simulink model "KD_cl_harness_cl_ouports_added"  (R2015b)
settings: Solver=ode45  StartTime=0  StopTime=inf  FixedStep=0.01  MaxStep=0.005  RelTol=1e-5  AbsTol=1e-5
undefined symbols (not defined in the file or in its folder): A2, bin_vec, c_0, c_1000, c_1000inv, c_100inv, c_1d2p4, c_1p7, c_4400inv, c_5500inv, c_80, c_compmap, c_ctok, c_fflow_max, c_fflow_min, c_filt, c_flowdiv, c_flowmin, c_flowmult, c_inf, c_km1d2k, c_n1, c_p00001, c_p01, c_p1e9, c_p4d1p4, c_pincomp, c_rair, c_roacorr, c_rpmtoradpers, c_svrthrottle1, c_svrthrottle2, c_svrthrottlearg, c_svrthrottlebeta, c_vnliftmax, c_vnliftmin, cl_offset, clff, Coefs, const, const_exhat, const_vec, Dual_array, dual_zero, egr_ecu_ff, expcon, f_mat, gs_jul, HQP_eps, HQP_INF, HQP_saturation, IV, L2, length_L, maxL, mHQP_saturation, minL, Newton, nRed, num_constraints ... (+22)
libraries: simulink x33
(part 1 of 6)
settings Model: Creator=spolavarapu  LastModifiedBy=rthekkal
settings SolverCC: ZeroCrossControl=DisableAll
settings DataIOCC: LimitDataPoints=off  SaveFormat=StructureWithTime  SignalLoggingSaveFormat=ModelDataLogs  SaveOutput=off  SignalLogging=off  DSMLogging=off  SaveTime=off
settings OptimizationCC: BlockReduction=off  OptimizeBlockIOStorage=off  BufferReuse=off  GlobalBufferReuse=off  ExpressionFolding=off  ExpressionDepthLimit=2147483647  LocalBlockOutputs=off  EfficientFloat2IntCast=on  OptimizeModelRefInitCode=on
settings DebuggingCC: SignalInfNanChecking=error  SignalRangeChecking=error  ReadBeforeWriteMsg=DisableAll  WriteAfterWriteMsg=DisableAll  WriteAfterReadMsg=DisableAll  AlgebraicLoopMsg=error  ArtificialAlgebraicLoopMsg=error  SaveWithDisabledLinksMsg=error  SaveWithParameterizedLinksMsg=error  UnderspecifiedInitializationDetection=Classic  MergeDetectMultiDrivingBlocksExec=none  CheckExecutionContextPreStartOutputMsg=on  CheckExecutionContextRuntimeOutputMsg=on  BlockPriorityViolationMsg=error  SolverPrmCheckMsg=error  InheritedTsInSrcMsg=error  MultiTaskDSMMsg=none  SigSpecEnsureSampleTimeMsg=error  CheckMatrixSingularityMsg=error  IntegerOverflowMsg=error  ParameterUnderflowMsg=error  ParameterPrecisionLossMsg=error  ParameterTunabilityLossMsg=error  UnderSpecifiedDataTypeMsg=warning  UnnecessaryDatatypeConvMsg=warning  VectorMatrixConversionMsg=error  FcnCallInpInsideContextMsg=EnableAllAsWarning  SignalLabelMismatchMsg=warning  UnconnectedInputMsg=error  UnconnectedOutputMsg=error  UnconnectedLineMsg=error  SFcnCompatibilityMsg=error  UniqueDataStoreMsg=error  BusObjectLabelMismatch=error  RootOutportRequireBusObject=error  AssertControl=DisableAll  ModelReferenceIOMsg=error  ModelReferenceIOMismatchMessage=error  UnknownTsInhSupMsg=error  ModelReferenceDataLoggingMessage=error  StateNameClashWarn=warning  StrictBusMsg=ErrorOnBusTreatedAsVector  IntegerSaturationMsg=error
settings HardwareCC: ProdBitPerPointer=32  ProdLargestAtomicFloat=None  ProdIntDivRoundTo=Undefined  ProdEndianess=Unspecified  ProdWordSize=32  ProdHWDeviceType=32-bit Generic
settings RTWCC: SystemTargetFile=ert.tlc  TemplateMakefile=ert_default_tmf  Description=Real-Time Workshop Embedded Coder
settings CodeAppCC: ForceParamTrailComments=on  IgnoreCustomStorageClasses=off  MangleLength=4  CustomSymbolStrType=$N$R$M  InternalIdentifier=Classic  ReqsInCode=on
settings ERTTargetCC: GenerateSampleERTMain=on  IncludeMdlTerminateFcn=off  GeneratePreprocessorConditionals=Disable all  SuppressErrorStatus=on  SupportAbsoluteTime=off  SupportNonFinite=off  ParenthesesLevel=Maximum  ERTCustomFileTemplate=example_file_process.tlc  PreserveExpressionOrder=on  PreserveIfCondition=on
settings ConfigComp: CovModelRefEnable=Off

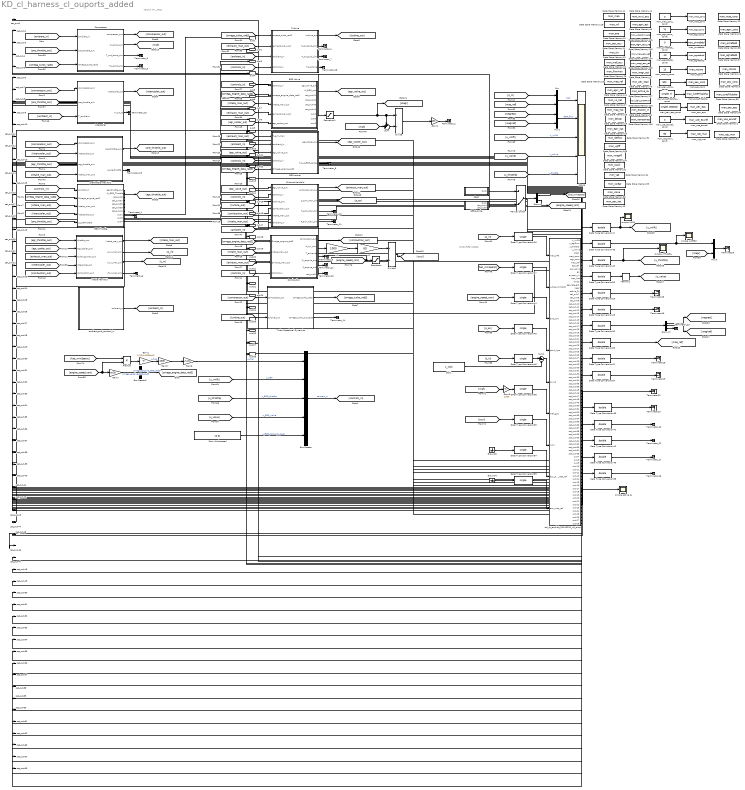
== system KD_cl_harness_cl_ouports_added ==
  note: Version A4 _ 0611
  note: SIMPLIFIED MODEL
  Bus Creator : BusCreator  Inputs=5
  Bus Creator2 : BusCreator  Inputs=1
  Combsution : Subsystem
  Compressor : Subsystem
  Data Store Memory10 : DataStoreMemory  DataStoreName=mon_ene  ReadBeforeWriteMsg=warning  WriteAfterWriteMsg=warning  WriteAfterReadMsg=warning  InitialValue=1  OutDataTypeStr=single
  Data Store Memory100 : DataStoreMemory  DataStoreName=mon_remapmap  ReadBeforeWriteMsg=warning  WriteAfterWriteMsg=warning  WriteAfterReadMsg=warning  OutDataTypeStr=single
  Data Store Memory103 : DataStoreMemory  DataStoreName=mon_egrr_ecu_ref  ReadBeforeWriteMsg=warning  WriteAfterWriteMsg=warning  WriteAfterReadMsg=warning  InitialValue=1  OutDataTypeStr=single
  Data Store Memory104 : DataStoreMemory  DataStoreName=mon_map_ecu_ref  ReadBeforeWriteMsg=warning  WriteAfterWriteMsg=warning  WriteAfterReadMsg=warning  InitialValue=1  OutDataTypeStr=single
  Data Store Memory105 : DataStoreMemory  DataStoreName=mon_wegr_ecu_ref  ReadBeforeWriteMsg=warning  WriteAfterWriteMsg=warning  WriteAfterReadMsg=warning  InitialValue=1  OutDataTypeStr=single
  Data Store Memory106 : DataStoreMemory  DataStoreName=mon_wtpostinverse  ReadBeforeWriteMsg=warning  WriteAfterWriteMsg=warning  WriteAfterReadMsg=warning  InitialValue=1  OutDataTypeStr=single
  Data Store Memory107 : DataStoreMemory  DataStoreName=mon_vwegrff  ReadBeforeWriteMsg=warning  WriteAfterWriteMsg=warning  WriteAfterReadMsg=warning  InitialValue=1  OutDataTypeStr=single
  Data Store Memory108 : DataStoreMemory  DataStoreName=mon_vgtff  ReadBeforeWriteMsg=warning  WriteAfterWriteMsg=warning  WriteAfterReadMsg=warning  InitialValue=1  OutDataTypeStr=single
  Data Store Memory11 : DataStoreMemory  DataStoreName=mon_pex_ecu  ReadBeforeWriteMsg=warning  WriteAfterWriteMsg=warning  WriteAfterReadMsg=warning  InitialValue=1  OutDataTypeStr=single
  Data Store Memory118 : DataStoreMemory  DataStoreName=mon_wf  ReadBeforeWriteMsg=warning  WriteAfterWriteMsg=warning  WriteAfterReadMsg=warning  InitialValue=1  OutDataTypeStr=single
  Data Store Memory126 : DataStoreMemory  DataStoreName=mon_delU_HQPKWIK  ReadBeforeWriteMsg=warning  WriteAfterWriteMsg=warning  WriteAfterReadMsg=warning  InitialValue=[0;0;0]  OutDataTypeStr=single
  Data Store Memory127 : DataStoreMemory  DataStoreName=mon_active_SL  ReadBeforeWriteMsg=warning  WriteAfterWriteMsg=warning  WriteAfterReadMsg=warning  OutDataTypeStr=int32
  Data Store Memory13 : DataStoreMemory  DataStoreName=mon_tin  ReadBeforeWriteMsg=warning  WriteAfterWriteMsg=warning  WriteAfterReadMsg=warning  InitialValue=1  OutDataTypeStr=single
  Data Store Memory14 : DataStoreMemory  DataStoreName=man_ntcons  ReadBeforeWriteMsg=warning  WriteAfterWriteMsg=warning  WriteAfterReadMsg=warning  InitialValue=15  OutDataTypeStr=single
  Data Store Memory2 : DataStoreMemory  DataStoreName=man_use_ecuref  ReadBeforeWriteMsg=warning  WriteAfterWriteMsg=warning  WriteAfterReadMsg=warning  OutDataTypeStr=single
  Data Store Memory20 : DataStoreMemory  DataStoreName=mon_maf_ecu  ReadBeforeWriteMsg=warning  WriteAfterWriteMsg=warning  WriteAfterReadMsg=warning  InitialValue=1  OutDataTypeStr=single
  Data Store Memory21 : DataStoreMemory  DataStoreName=man_map_cons  ReadBeforeWriteMsg=warning  WriteAfterWriteMsg=warning  WriteAfterReadMsg=warning  OutDataTypeStr=single
  Data Store Memory22 : DataStoreMemory  DataStoreName=man_egrr_cons  ReadBeforeWriteMsg=warning  WriteAfterWriteMsg=warning  WriteAfterReadMsg=warning  InitialValue=70  OutDataTypeStr=single
  Data Store Memory23 : DataStoreMemory  DataStoreName=mon_map_ref  ReadBeforeWriteMsg=warning  WriteAfterWriteMsg=warning  WriteAfterReadMsg=warning  InitialValue=1  OutDataTypeStr=single
  Data Store Memory24 : DataStoreMemory  DataStoreName=mon_egrr_ref  ReadBeforeWriteMsg=warning  WriteAfterWriteMsg=warning  WriteAfterReadMsg=warning  InitialValue=1  OutDataTypeStr=single
  Data Store Memory25 : DataStoreMemory  DataStoreName=mon_map_hat  ReadBeforeWriteMsg=warning  WriteAfterWriteMsg=warning  WriteAfterReadMsg=warning  InitialValue=1  OutDataTypeStr=single
  Data Store Memory26 : DataStoreMemory  DataStoreName=mon_egrr_hat  ReadBeforeWriteMsg=warning  WriteAfterWriteMsg=warning  WriteAfterReadMsg=warning  InitialValue=1  OutDataTypeStr=single
  Data Store Memory27 : DataStoreMemory  DataStoreName=mon_x1_hat  ReadBeforeWriteMsg=warning  WriteAfterWriteMsg=warning  WriteAfterReadMsg=warning  InitialValue=zeros(nRed,1)  OutDataTypeStr=single
  Data Store Memory28 : DataStoreMemory  DataStoreName=mon_flowmax  ReadBeforeWriteMsg=warning  WriteAfterWriteMsg=warning  WriteAfterReadMsg=warning  InitialValue=1  OutDataTypeStr=single
  Data Store Memory29 : DataStoreMemory  DataStoreName=mon_delvgt  ReadBeforeWriteMsg=warning  WriteAfterWriteMsg=warning  WriteAfterReadMsg=warning  InitialValue=1  OutDataTypeStr=single
  Data Store Memory31 : DataStoreMemory  DataStoreName=mon_delflow  ReadBeforeWriteMsg=warning  WriteAfterWriteMsg=warning  WriteAfterReadMsg=warning  InitialValue=1  OutDataTypeStr=single
  Data Store Memory32 : DataStoreMemory  DataStoreName=mon_slack  ReadBeforeWriteMsg=warning  WriteAfterWriteMsg=warning  WriteAfterReadMsg=warning  InitialValue=1  OutDataTypeStr=single
  Data Store Memory34 : DataStoreMemory  DataStoreName=mon_vgt  ReadBeforeWriteMsg=warning  WriteAfterWriteMsg=warning  WriteAfterReadMsg=warning  InitialValue=1  OutDataTypeStr=single
  Data Store Memory35 : DataStoreMemory  DataStoreName=mon_uwegr  ReadBeforeWriteMsg=warning  WriteAfterWriteMsg=warning  WriteAfterReadMsg=warning  InitialValue=1  OutDataTypeStr=single
  Data Store Memory36 : DataStoreMemory  DataStoreName=mon_valve  ReadBeforeWriteMsg=warning  WriteAfterWriteMsg=warning  WriteAfterReadMsg=warning  InitialValue=1  OutDataTypeStr=single
  Data Store Memory37 : DataStoreMemory  DataStoreName=man_egrrefadd  ReadBeforeWriteMsg=warning  WriteAfterWriteMsg=warning  WriteAfterReadMsg=warning  InitialValue=-10  OutDataTypeStr=single
  Data Store Memory38 : DataStoreMemory  DataStoreName=man_pinrefadd  ReadBeforeWriteMsg=warning  WriteAfterWriteMsg=warning  WriteAfterReadMsg=warning  OutDataTypeStr=single
  Data Store Memory41 : DataStoreMemory  DataStoreName=mon_map  ReadBeforeWriteMsg=warning  WriteAfterWriteMsg=warning  WriteAfterReadMsg=warning  InitialValue=1  OutDataTypeStr=single
  Data Store Memory43 : DataStoreMemory  DataStoreName=mon_pex_hat  ReadBeforeWriteMsg=warning  WriteAfterWriteMsg=warning  WriteAfterReadMsg=warning  InitialValue=3  OutDataTypeStr=single
  Data Store Memory44 : DataStoreMemory  DataStoreName=mon_wcyl_ecu  ReadBeforeWriteMsg=warning  WriteAfterWriteMsg=warning  WriteAfterReadMsg=warning  InitialValue=1  OutDataTypeStr=single
  Data Store Memory46 : DataStoreMemory  DataStoreName=mon_egrr_est  ReadBeforeWriteMsg=warning  WriteAfterWriteMsg=warning  WriteAfterReadMsg=warning  InitialValue=1  OutDataTypeStr=single
  Data Store Memory47 : DataStoreMemory  DataStoreName=mon_wegr_est  ReadBeforeWriteMsg=warning  WriteAfterWriteMsg=warning  WriteAfterReadMsg=warning  InitialValue=1  OutDataTypeStr=single
  Data Store Memory54 : DataStoreMemory  DataStoreName=man_pex_eps  ReadBeforeWriteMsg=warning  WriteAfterWriteMsg=warning  WriteAfterReadMsg=warning  InitialValue=single(.000002)  OutDataTypeStr=single
  Data Store Memory78 : DataStoreMemory  DataStoreName=mon_pex_lead  ReadBeforeWriteMsg=warning  WriteAfterWriteMsg=warning  WriteAfterReadMsg=warning  OutDataTypeStr=single
  Data Store Memory84 : DataStoreMemory  DataStoreName=man_vgt_max  ReadBeforeWriteMsg=warning  WriteAfterWriteMsg=warning  WriteAfterReadMsg=warning  InitialValue=90  OutDataTypeStr=single
  Data Store Memory85 : DataStoreMemory  DataStoreName=man_tuneFiltalpha  ReadBeforeWriteMsg=warning  WriteAfterWriteMsg=warning  WriteAfterReadMsg=warning  InitialValue=single(.7)  OutDataTypeStr=single
  Data Store Memory9 : DataStoreMemory  DataStoreName=man_pex_cons  ReadBeforeWriteMsg=warning  WriteAfterWriteMsg=warning  WriteAfterReadMsg=warning  InitialValue=300  OutDataTypeStr=single
  Data Store Memory91 : DataStoreMemory  DataStoreName=mon_expcon_in  ReadBeforeWriteMsg=warning  WriteAfterWriteMsg=warning  WriteAfterReadMsg=warning  InitialValue=zeros(nRed+12,1)  OutDataTypeStr=single
  Data Type Conversion{26,35,37..38,44..46,53..54} (9 alike) : DataTypeConversion  OutDataTypeStr=single
  Data Type Conversion{28..31,33..34,39,41..43,47..50,55} (15 alike) : DataTypeConversion  OutDataTypeStr=double
  Demux : Demux  Outputs=2
  Demux2 : Demux  Outputs=3
  Divide : Product  Inputs=*/
  Divide1 : Product  Inputs=*/
  EGR Throttle : Subsystem
  EGR Valve : Subsystem
  EGR cooler : Subsystem
  Exhaust Manifold : Subsystem
  From Workspace4 : FromWorkspace  VariableName=[0 3]  SampleTime=0  Interpolate=off  OutputAfterFinalValue=Holding final value
  Gain1 : Gain  Gain=1/(120/4/832e-9)
  Gain2 : Gain  Gain=100
  Gain5 : Gain  Gain=1000
  Gain6 : Gain  Gain=1/1000
  Gain7 : Gain  Gain=pi/30
  Gain9 : Gain  Gain=1000
  Ground3 : Ground
  Ground4 : Ground
  Intake Manifold : Subsystem
  Intercooler : Subsystem
  Manual Switch : ManualSwitch  CurrentSetting=0
  Memory1 : Memory
  Mux : Mux  Inputs=2
  Mux1 : Mux  Inputs=2
  Mux3 : Mux  Inputs=2
  NEDC_cycle : Subsystem
  Product : Product  RndMeth=Zero
  Saturation : Saturate  UpperLimit=6000  LowerLimit=500
  Saturation1 : Saturate  UpperLimit=inf  LowerLimit=0
      settings: AttributesFormatString=%<LowerLimit>\n%<UpperLimit>
  Scope : Scope  NumInputPorts=5
  Sum : Sum  Inputs=++|
  Sum1 : Sum  Inputs=|+-
  Terminator{5,12..13,15..16,18..19} (7 alike) : Terminator
  Terminator_{1..9,11,13..23,26} (22 alike) : Terminator
  Turbine : Subsystem
  Turbo Rotational Dynamics : Subsystem
  ambient_and_controls_in : Subsystem
  ctok1 : Constant  Value=c_ctok  OutDataTypeStr=single  SampleTime=sample_time
      settings: AttributesFormatString=%<Value>\n%<SampleTime>
  ctrl_rb_explicit_20140220_v6_simp : Subsystem  TreatAsAtomicUnit=on  SystemSampleTime=sample_time
  man_egrr_cons : DataStoreWrite  DataStoreName=man_egrr_cons
  man_egrr_cons_const : Constant  Value=70  OutDataTypeStr=single
  man_egrrefadd : DataStoreWrite  DataStoreName=man_egrrefadd
  man_egrrefadd_const : Constant  Value=-10  VectorParams1D=off  OutDataTypeStr=single
      settings: AttributesFormatString=%<VectorParams1D>
  man_map_cons : DataStoreWrite  DataStoreName=man_map_cons
  man_map_cons_const : Constant  Value=0  OutDataTypeStr=single
  man_ntcons : DataStoreWrite  DataStoreName=man_ntcons
  man_ntcons_const : Constant  Value=15  OutDataTypeStr=single
  man_pex_cons : DataStoreWrite  DataStoreName=man_pex_cons
  man_pex_cons_const : Constant  Value=300  OutDataTypeStr=single
  man_pex_eps : DataStoreWrite  DataStoreName=man_pex_eps
  man_pex_eps_const : Constant  Value=single(.000002)  OutDataTypeStr=single
  man_pinrefadd : DataStoreWrite  DataStoreName=man_pinrefadd
  man_pinrefadd_const : Constant  Value=0  OutDataTypeStr=single
  man_tuneFiltalpha : DataStoreWrite  DataStoreName=man_tuneFiltalpha
  man_tuneFiltalpha_const : Constant  Value=single(.7)  OutDataTypeStr=single
  man_use_ecuref : DataStoreWrite  DataStoreName=man_use_ecuref
  man_use_ecuref_const : Constant  Value=0  OutDataTypeStr=single
  man_vgt_max : DataStoreWrite  DataStoreName=man_vgt_max
  man_vgt_max_const : Constant  Value=90  OutDataTypeStr=single
  n1 : Gain  Gain=1000
      settings: AttributesFormatString=%<Gain>
  n2 : Gain  Gain=60
      settings: AttributesFormatString=%<Gain>
  pre-throttle manifold : Subsystem
  simple VNlift : Scope
  simple active SL : Scope
  simple uThrottle : Scope
  simple uWEGR : Scope
  steps : Subsystem
  sat_out-1 : Outport
  sat_out-2 : Outport  Port=2
  sat_out-3 : Outport  Port=3
  sat_out-4 : Outport  Port=4
  sat_out-5 : Outport  Port=5
  sat_out-6 : Outport  Port=6
  sat_out-7 : Outport  Port=7
  sat_out-8 : Outport  Port=8
  sat_out-9 : Outport  Port=9
  sat_out-10 : Outport  Port=10
  sat_out-11 : Outport  Port=11
  sat_out-12 : Outport  Port=12
  sat_out-13 : Outport  Port=13
  sat_out-14 : Outport  Port=14
  sat_out-15 : Outport  Port=15
  sat_out-16 : Outport  Port=16
  sat_out-17 : Outport  Port=17
  sat_out-18 : Outport  Port=18
  sat_out-19 : Outport  Port=19
  sat_out-20 : Outport  Port=20
  sat_out-21 : Outport  Port=21
  sat_out-22 : Outport  Port=22
  sat_out-23 : Outport  Port=23
  sat_out-24 : Outport  Port=24
  sat_out-25 : Outport  Port=25
  sat_out-26 : Outport  Port=26
  sat_out-27 : Outport  Port=27
  sat_out-28 : Outport  Port=28
  sat_out-29 : Outport  Port=29
  sat_out-30 : Outport  Port=30
  sat_out-31 : Outport  Port=31
  sat_out-32 : Outport  Port=32
  sat_out-33 : Outport  Port=33
  sat_out-34 : Outport  Port=34
  sat_out-35 : Outport  Port=35
  sat_out-36 : Outport  Port=36
  sat_out-37 : Outport  Port=37
  sat_out-38 : Outport  Port=38
  sat_out-39 : Outport  Port=39
  sat_out-40 : Outport  Port=40
  sat_out-41 : Outport  Port=41
  sat_out-42 : Outport  Port=42
  sat_out-43 : Outport  Port=43
  sat_out-44 : Outport  Port=44
  sat_out-45 : Outport  Port=45
  sat_out-46 : Outport  Port=46
  sat_out-47 : Outport  Port=47
  sat_out-48 : Outport  Port=48
  sat_out-49 : Outport  Port=49
  sat_out-50 : Outport  Port=50
  sat_out-51 : Outport  Port=51
  sat_out-52 : Outport  Port=52
  sat_out-53 : Outport  Port=53
  sat_out-54 : Outport  Port=54
  sat_out-55 : Outport  Port=55
  sat_out-56 : Outport  Port=56
  sat_out-57 : Outport  Port=57
  sat_out-58 : Outport  Port=58
  sat_out-59 : Outport  Port=59
  sat_out-60 : Outport  Port=60
  sat_out-61 : Outport  Port=61
  sat_out-62 : Outport  Port=62
  sat_out-63 : Outport  Port=63
  sat_out-64 : Outport  Port=64
  sat_out-65 : Outport  Port=65
  out-1 : Outport  Port=66
  out-2 : Outport  Port=67
  out-3 : Outport  Port=68
  out-4 : Outport  Port=69
  out-5 : Outport  Port=70
  out-6 : Outport  Port=71
  out-7 : Outport  Port=72
  out-8 : Outport  Port=73
  out-9 : Outport  Port=74
  out-10 : Outport  Port=75
  out-11 : Outport  Port=76
  out-12 : Outport  Port=77
  out-13 : Outport  Port=78
  out-14 : Outport  Port=79
  out-15 : Outport  Port=80
  out-16 : Outport  Port=81
  out-17 : Outport  Port=82
  out-18 : Outport  Port=83
  out-19 : Outport  Port=84
  out-20 : Outport  Port=85
  out-21 : Outport  Port=86
  out-22 : Outport  Port=87
  out-23 : Outport  Port=88
  out-24 : Outport  Port=89
  out-25 : Outport  Port=90
  out-26 : Outport  Port=91
  out-27 : Outport  Port=92
  out-28 : Outport  Port=93
  wires:
  ambient_and_controls_in/1(ambient_in) -> [ambient_in]
  Compressor/1(compressor_out) -> [compressor_out]
  Intercooler/1(intercooler_out) -> [intercooler_out]
  EGR Throttle/1(egr_throttle_out) -> [egr_throttle_out]
  Intake Manifold/1(intake_man_out) -> [intake_man_out]
  Turbine/1(turbine_out) -> [turbine_out]
  EGR Valve/1(egr_valve_out) -> [egr_valve_out]
  EGR cooler/1(egr_cooler_out) -> [egr_cooler_out]
  Exhaust Manifold/1(exhaust_man_out) -> [exhaust_man_out]
  Combsution/1(combustion_out) -> [combustion_out]
  pre-throttle manifold/1(pre_throttle_out) -> [pre_throttle_out]
  Compressor/2(W_comp_sim) -> [maf]
  Compressor/3(T_out_comp_sim) -> Terminator_3/1
  Compressor/4(Tq_comp_sim) -> Terminator_5/1
  EGR Valve/2(W_EGR_out) -> Saturation1/1, sat_out-2/1
  Exhaust Manifold/4(F_exh_man_sim) -> Terminator_11/1
  Intake Manifold/3(T_in_man_sim) -> [t_in]
  Intercooler/2(T_out_IC) -> Terminator_15/1
  Turbine/4(Tq_turbine) -> Terminator_18/1
  pre-throttle manifold/2(p_pre_throttle) -> Terminator_19/1
  Turbo Rotational Dynamics/1(Omega_turbo_radS) -> [omega_turbo_radS]
  Combsution/4(W_engine_out) -> Terminator_21/1
  Combsution/5(F_engine_out) -> Terminator_20/1
  Intake Manifold/2(p_in_man_sim) -> [p_in]
  Turbo Rotational Dynamics/2(Omega_turbo_out_radS) -> Terminator_14/1
  [maf] -> Sum/2
  Sum/1 -> Divide/2
  Divide/1 -> Gain2/1
  Exhaust Manifold/2(p_exh_man_sim) -> [p_ex]
  Turbine/2(W_out_turb_sim) -> Terminator_4/1
  Turbine/3(T_out_turb_sim) -> Terminator_7/1
  [p_in] -> Mux/1
  [u_vnlift] -> Bus Creator/2  "u_VGT"
  [u_throttle] -> Bus Creator/3  "u_EGR_throttle"
  [u_valve] -> Bus Creator/4  "u_EGR_valve"
  From Workspace4/1 -> Bus Creator/5  "u_EGR_cooler_bypass"
  Bus Creator/1 -> [controls_in]  "controls_in"
  Bus Creator2/1 -> [omega_engine_data_radS]  "omega_engine_data_radS"
  Mux/1 -> Scope/1  "MAP"
  Mux1/1 -> Scope/2  "EGR_flow"
  [map_ref] -> Mux/2
  Gain2/1 -> Terminator_2/1
  Exhaust Manifold/3(T_exh_man_sim) -> Terminator_16/1
  Gain7/1 -> Bus Creator2/1  "omega_engine_data_radS"
  [engine_speed_rpm] -> Gain7/1, Product/2
  [u_vnlift] -> Scope/3  "u_vnlift"
  [u_valve] -> Scope/4  "u_valve"
  EGR Throttle/2(W_EGR_Throttle) -> Terminator_1/1
  Saturation1/1 -> Sum/1, Divide/1, [Wegr]
  [ambient_in] -> Compressor/1(ambient_in)
  [compressor_out] -> Intercooler/1(compressor_out)
  [compressor_out] -> pre-throttle manifold/1(compressor_out)
  [intercooler_out] -> pre-throttle manifold/2(intercooler_out)
  [egr_throttle_out] -> pre-throttle manifold/3(egr_throttle_out)
  [controls_in] -> EGR Throttle/1(controls_in)
  [omega_engine_data_radS] -> EGR Throttle/2(Omega_engine_radS)
  [intake_man_out] -> EGR Throttle/3(intake_man_out)
  [intercooler_out] -> EGR Throttle/4(intercooler_out)
  [egr_throttle_out] -> Intake Manifold/1(throttle_out)
  [egr_cooler_out] -> Intake Manifold/2(egr_cooler_out)
  [exhaust_man_out] -> Intake Manifold/3(exhaust_man_out)
  [omega_turbo_radS] -> Compressor/3(Omega_turbo_radS)
  [pre_throttle_out] -> Compressor/2(pre_throttle_out)
  [pre_throttle_out] -> Intercooler/2(pre_throttle_out)
  [intercooler_out] -> Intake Manifold/4(intecooler_out)
  [combustion_out] -> Intake Manifold/5(combustion_out)
  [pre_throttle_out] -> EGR Throttle/5(p_preThrottle)
  [intake_man_out] -> pre-throttle manifold/4(Intake_man_out)
  [ambient_in] -> Intercooler/3(T_ambient)
  [omega_engine_data_radS] -> Combsution/1(Omega_engine_radS)
  [intake_man_out] -> Combsution/2(intake_man_out)
  [exhaust_man_out] -> Combsution/3(exhaust_man_out)
  [controls_in] -> Combsution/4(controls_in)
  [intake_man_out] -> Exhaust Manifold/5(intake_man_out)
  [egr_valve_out] -> Exhaust Manifold/1(egr_valve_out)
  [controls_in] -> Exhaust Manifold/2(controls_in)
  [turbine_out] -> Exhaust Manifold/3(turbine_out)
  [ambient_in] -> EGR cooler/2(ambient_in)
  [exhaust_man_out] -> EGR cooler/1(T_exh_man)
  [egr_valve_out] -> EGR cooler/3(egr_valve_out)
  [controls_in] -> EGR cooler/4(controls_in)
  [omega_engine_data_radS] -> EGR cooler/5(Omega_engine_radS)
  [exhaust_man_out] -> EGR Valve/4(exhaust_man_out)
  [controls_in] -> EGR Valve/1(controls_in)
  [omega_engine_data_radS] -> EGR Valve/2(omega_engine_data_radS)
  [intake_man_out] -> EGR Valve/3(intake_man_out)
  [omega_turbo_radS] -> Turbine/1(omega_turbo_radS)
  [exhaust_man_out] -> Turbine/2(exhaust_man_out)
  [ambient_in] -> Turbine/3(ambient_In)
  [controls_in] -> Turbine/4(controls_In)
  [compressor_out] -> Turbo Rotational Dynamics/1(compressor_out)
  [turbine_out] -> Turbo Rotational Dynamics/2(turbine_out)
  [combustion_out] -> Exhaust Manifold/4(combustion_out)
  [egr_cooler_out] -> EGR Valve/5(egr_cooler_out)
  [ambient_in] -> Exhaust Manifold/6(ambient_in)
  Intake Manifold/4(F_in_man_sim) -> Terminator_6/1
  Combsution/3(T_exhaust) -> Terminator_9/1
  Product/1 -> Gain1/1
  [fuel_mm3perst] -> Product/1
  [u_throttle] -> Scope/5  "u_throttle"
  NEDC_cycle/1(Out1) -> Manual Switch/2
  steps/1(Out1) -> Manual Switch/1
  Manual Switch/1 -> Demux/1
  Demux/1 -> [fuel_mm3perst]
  Demux/2 -> [engine_speed_rpm]
  EGR cooler/2(T_out_EGR_cooler) -> Terminator_8/1
  Gain5/1 -> Gain6/1
  Gain6/1 -> Bus Creator/1  "u_fuel"
  Gain1/1 -> Gain5/1  "u_fuel"
  Combsution/2(W_cyl_sim) -> n1/1
  n1/1 -> n2/1
  n2/1 -> Divide1/1
  [engine_speed_rpm] -> Saturation/1, sat_out-1/1
  Divide1/1 -> [wcyl]
  Saturation/1 -> Divide1/2
  ctrl_rb_explicit_20140220_v6_simp/3(u_throttle) -> Data Type Conversion49/1
  ctrl_rb_explicit_20140220_v6_simp/2(u_egrflow) -> Data Type Conversion48/1
  ctrl_rb_explicit_20140220_v6_simp/4(u_valve) -> Data Type Conversion50/1
  ctrl_rb_explicit_20140220_v6_simp/5(slack) -> Data Type Conversion28/1
  ctrl_rb_explicit_20140220_v6_simp/6(map_cons) -> Data Type Conversion29/1
  ctrl_rb_explicit_20140220_v6_simp/7(egr_cons) -> Data Type Conversion30/1
  ctrl_rb_explicit_20140220_v6_simp/1(u_vnlift) -> Data Type Conversion47/1
  [p_in] -> Data Type Conversion26/1
  [fuel_mm3perst] -> Data Type Conversion37/1
  [engine_speed_rpm] -> Data Type Conversion44/1
  [p_ex] -> Data Type Conversion45/1
  [t_in] -> Data Type Conversion46/1
  ctrl_rb_explicit_20140220_v6_simp/8(map_ref) -> Data Type Conversion33/1
  Data Type Conversion49/1 -> simple uThrottle/1, [u_throttle]
  Data Type Conversion50/1 -> Memory1/1
  Data Type Conversion28/1 -> Terminator15/1
  Data Type Conversion29/1 -> Terminator16/1
  Data Type Conversion30/1 -> Demux2/1
  Data Type Conversion33/1 -> [map_ref]
  ctrl_rb_explicit_20140220_v6_simp/9(egr_ref) -> Data Type Conversion31/1
  Data Type Conversion31/1 -> Terminator18/1
  ctrl_rb_explicit_20140220_v6_simp/10(pex_cons) -> Data Type Conversion34/1
  Data Type Conversion34/1 -> Terminator19/1
  Data Type Conversion48/1 -> Mux3/1, simple uWEGR/1
  Mux3/1 -> Terminator5/1
  [Wegr] -> Mux3/2
  ctrl_rb_explicit_20140220_v6_simp/11(gs) -> Terminator12/1
  Data Type Conversion26/1 -> ctrl_rb_explicit_20140220_v6_simp/1(map_kPa)
  Data Type Conversion37/1 -> ctrl_rb_explicit_20140220_v6_simp/2(u_fuel_mm3pst)
  Data Type Conversion44/1 -> ctrl_rb_explicit_20140220_v6_simp/3(ene_rpm)
  Data Type Conversion45/1 -> ctrl_rb_explicit_20140220_v6_simp/4(pexh_kpa)
  Memory1/1 -> [u_valve]
  Data Type Conversion39/1 -> Terminator13/1
  Gain9/1 -> Data Type Conversion38/1
  [maf] -> Gain9/1
  Data Type Conversion38/1 -> ctrl_rb_explicit_20140220_v6_simp/6(maf_gps)
  Data Type Conversion46/1 -> Sum1/1
  ctok1/1 -> Sum1/2
  Sum1/1 -> ctrl_rb_explicit_20140220_v6_simp/5(t_in_C)
  [wcyl] -> Data Type Conversion35/1
  Data Type Conversion35/1 -> ctrl_rb_explicit_20140220_v6_simp/7(wcyl)
  ctrl_rb_explicit_20140220_v6_simp/13(pex_hat) -> Data Type Conversion41/1
  ctrl_rb_explicit_20140220_v6_simp/14(dwdp) -> Data Type Conversion42/1
  Data Type Conversion42/1 -> Terminator_22/1
  Data Type Conversion41/1 -> Terminator_13/1
  ctrl_rb_explicit_20140220_v6_simp/15(egr_rate_est) -> Data Type Conversion43/1
  Data Type Conversion43/1 -> Terminator_17/1
  ctrl_rb_explicit_20140220_v6_simp/17(active_SL) -> simple active SL/1
  Demux2/3 -> Terminator_23/1
  Demux2/2 -> [wegrref]
  Demux2/1 -> [wegrest]
  Data Type Conversion47/1 -> simple VNlift/1, [u_vnlift]
  Data Type Conversion54/1 -> ctrl_rb_explicit_20140220_v6_simp/8(ecu_egr_rate_ref)
  Data Type Conversion53/1 -> ctrl_rb_explicit_20140220_v6_simp/9(ecu_map_ref)
  Ground3/1 -> Data Type Conversion54/1
  Ground4/1 -> Data Type Conversion53/1
  ctrl_rb_explicit_20140220_v6_simp/16(wegr) -> Data Type Conversion55/1
  Data Type Conversion55/1 -> Terminator_26/1
  ctrl_rb_explicit_20140220_v6_simp/12(expcon_in) -> Data Type Conversion39/1
  man_map_cons_const/1 -> man_map_cons/1
  man_egrr_cons_const/1 -> man_egrr_cons/1
  man_pinrefadd_const/1 -> man_pinrefadd/1
  man_egrrefadd_const/1 -> man_egrrefadd/1
  man_ntcons_const/1 -> man_ntcons/1
  man_pex_cons_const/1 -> man_pex_cons/1
  man_tuneFiltalpha_const/1 -> man_tuneFiltalpha/1
  man_pex_eps_const/1 -> man_pex_eps/1
  man_vgt_max_const/1 -> man_vgt_max/1
  man_use_ecuref_const/1 -> man_use_ecuref/1
  [wegrest] -> Mux1/1
  [wegrref] -> Mux1/2
  Combsution/6(sat_out-3) -> sat_out-3/1
  NEDC_cycle/2(sat_out-4) -> sat_out-4/1
  NEDC_cycle/3(sat_out-5) -> sat_out-5/1
  EGR Throttle/3(sat_out-6) -> sat_out-6/1
  ctrl_rb_explicit_20140220_v6_simp/18(sat_out-7) -> sat_out-7/1
  ctrl_rb_explicit_20140220_v6_simp/19(sat_out-8) -> sat_out-8/1
  ctrl_rb_explicit_20140220_v6_simp/20(sat_out-9) -> sat_out-9/1
  ctrl_rb_explicit_20140220_v6_simp/21(sat_out-10) -> sat_out-10/1
  ctrl_rb_explicit_20140220_v6_simp/22(sat_out-11) -> sat_out-11/1
  ctrl_rb_explicit_20140220_v6_simp/23(sat_out-12) -> sat_out-12/1
  ctrl_rb_explicit_20140220_v6_simp/24(sat_out-13) -> sat_out-13/1
  ctrl_rb_explicit_20140220_v6_simp/25(sat_out-14) -> sat_out-14/1
  ctrl_rb_explicit_20140220_v6_simp/26(sat_out-15) -> sat_out-15/1
  ctrl_rb_explicit_20140220_v6_simp/27(sat_out-16) -> sat_out-16/1
  ctrl_rb_explicit_20140220_v6_simp/28(sat_out-17) -> sat_out-17/1
  ctrl_rb_explicit_20140220_v6_simp/29(sat_out-18) -> sat_out-18/1
  ctrl_rb_explicit_20140220_v6_simp/30(sat_out-19) -> sat_out-19/1
  ctrl_rb_explicit_20140220_v6_simp/31(sat_out-20) -> sat_out-20/1
  ctrl_rb_explicit_20140220_v6_simp/32(sat_out-21) -> sat_out-21/1
  ctrl_rb_explicit_20140220_v6_simp/33(sat_out-22) -> sat_out-22/1
  ctrl_rb_explicit_20140220_v6_simp/34(sat_out-23) -> sat_out-23/1
  ctrl_rb_explicit_20140220_v6_simp/35(sat_out-24) -> sat_out-24/1
  ctrl_rb_explicit_20140220_v6_simp/36(sat_out-25) -> sat_out-25/1
  ctrl_rb_explicit_20140220_v6_simp/37(sat_out-26) -> sat_out-26/1
  ctrl_rb_explicit_20140220_v6_simp/38(sat_out-27) -> sat_out-27/1
  ctrl_rb_explicit_20140220_v6_simp/39(sat_out-28) -> sat_out-28/1
  ctrl_rb_explicit_20140220_v6_simp/40(sat_out-29) -> sat_out-29/1
  ctrl_rb_explicit_20140220_v6_simp/41(sat_out-30) -> sat_out-30/1
  ctrl_rb_explicit_20140220_v6_simp/42(sat_out-31) -> sat_out-31/1
  ctrl_rb_explicit_20140220_v6_simp/43(sat_out-32) -> sat_out-32/1
  ctrl_rb_explicit_20140220_v6_simp/44(sat_out-33) -> sat_out-33/1
  ctrl_rb_explicit_20140220_v6_simp/45(sat_out-34) -> sat_out-34/1
  ctrl_rb_explicit_20140220_v6_simp/46(sat_out-35) -> sat_out-35/1
  ctrl_rb_explicit_20140220_v6_simp/47(sat_out-36) -> sat_out-36/1
  EGR Throttle/4(sat_out-37) -> sat_out-37/1
  EGR Throttle/5(sat_out-38) -> sat_out-38/1
  EGR Throttle/6(sat_out-39) -> sat_out-39/1
  EGR Throttle/7(sat_out-40) -> sat_out-40/1
  EGR Valve/3(sat_out-41) -> sat_out-41/1
  EGR Valve/4(sat_out-42) -> sat_out-42/1
  EGR Valve/5(sat_out-43) -> sat_out-43/1
  EGR Valve/6(sat_out-44) -> sat_out-44/1
  ctrl_rb_explicit_20140220_v6_simp/48(sat_out-45) -> sat_out-45/1
  ctrl_rb_explicit_20140220_v6_simp/49(sat_out-46) -> sat_out-46/1
  ctrl_rb_explicit_20140220_v6_simp/50(sat_out-47) -> sat_out-47/1
  ctrl_rb_explicit_20140220_v6_simp/51(sat_out-48) -> sat_out-48/1
  ctrl_rb_explicit_20140220_v6_simp/52(sat_out-49) -> sat_out-49/1
  ctrl_rb_explicit_20140220_v6_simp/53(sat_out-50) -> sat_out-50/1
  ctrl_rb_explicit_20140220_v6_simp/54(sat_out-51) -> sat_out-51/1
  ctrl_rb_explicit_20140220_v6_simp/55(sat_out-52) -> sat_out-52/1
  ctrl_rb_explicit_20140220_v6_simp/56(sat_out-53) -> sat_out-53/1
  ctrl_rb_explicit_20140220_v6_simp/57(sat_out-54) -> sat_out-54/1
  ctrl_rb_explicit_20140220_v6_simp/58(sat_out-55) -> sat_out-55/1
  ctrl_rb_explicit_20140220_v6_simp/59(sat_out-56) -> sat_out-56/1
  ctrl_rb_explicit_20140220_v6_simp/60(sat_out-57) -> sat_out-57/1
  ctrl_rb_explicit_20140220_v6_simp/61(sat_out-58) -> sat_out-58/1
  ctrl_rb_explicit_20140220_v6_simp/62(sat_out-59) -> sat_out-59/1
  ctrl_rb_explicit_20140220_v6_simp/63(sat_out-60) -> sat_out-60/1
  ctrl_rb_explicit_20140220_v6_simp/64(sat_out-61) -> sat_out-61/1
  ctrl_rb_explicit_20140220_v6_simp/65(sat_out-62) -> sat_out-62/1
  ctrl_rb_explicit_20140220_v6_simp/66(sat_out-63) -> sat_out-63/1
  ctrl_rb_explicit_20140220_v6_simp/67(sat_out-64) -> sat_out-64/1
  ctrl_rb_explicit_20140220_v6_simp/68(sat_out-65) -> sat_out-65/1
  EGR Throttle/8(out-1) -> out-1/1
  EGR Valve/7(out-2) -> out-2/1
  EGR Throttle/9(out-3) -> out-3/1
  EGR Throttle/10(out-4) -> out-4/1
  EGR Valve/8(out-5) -> out-5/1
  EGR Valve/9(out-6) -> out-6/1
  ctrl_rb_explicit_20140220_v6_simp/69(out-7) -> out-7/1
  ctrl_rb_explicit_20140220_v6_simp/70(out-8) -> out-8/1
  ctrl_rb_explicit_20140220_v6_simp/71(out-9) -> out-9/1
  ctrl_rb_explicit_20140220_v6_simp/72(out-10) -> out-10/1
  ctrl_rb_explicit_20140220_v6_simp/73(out-11) -> out-11/1
  ctrl_rb_explicit_20140220_v6_simp/74(out-12) -> out-12/1
  ctrl_rb_explicit_20140220_v6_simp/75(out-13) -> out-13/1
  ctrl_rb_explicit_20140220_v6_simp/76(out-14) -> out-14/1
  ctrl_rb_explicit_20140220_v6_simp/77(out-15) -> out-15/1
  ctrl_rb_explicit_20140220_v6_simp/78(out-16) -> out-16/1
  ctrl_rb_explicit_20140220_v6_simp/79(out-17) -> out-17/1
  ctrl_rb_explicit_20140220_v6_simp/80(out-18) -> out-18/1
  ctrl_rb_explicit_20140220_v6_simp/81(out-19) -> out-19/1
  ctrl_rb_explicit_20140220_v6_simp/82(out-20) -> out-20/1
  ctrl_rb_explicit_20140220_v6_simp/83(out-21) -> out-21/1
  ctrl_rb_explicit_20140220_v6_simp/84(out-22) -> out-22/1
  ctrl_rb_explicit_20140220_v6_simp/85(out-23) -> out-23/1
  ctrl_rb_explicit_20140220_v6_simp/86(out-24) -> out-24/1
  ctrl_rb_explicit_20140220_v6_simp/87(out-25) -> out-25/1
  ctrl_rb_explicit_20140220_v6_simp/88(out-26) -> out-26/1
  ctrl_rb_explicit_20140220_v6_simp/89(out-27) -> out-27/1
  ctrl_rb_explicit_20140220_v6_simp/90(out-28) -> out-28/1

== system KD_cl_harness_cl_ouports_added/Combsution ==
  note: W_engine = W_cyl + u_fuel
  note: Gain block has no significance
      | just to add color to the lines
  Omega_engine_radS : Inport
  intake_man_out : Inport  Port=2
  exhaust_man_out : Inport  Port=3
  controls_in : Inport  Port=4
  Bus Creator : BusCreator  Inputs=4
  Bus Creator1 : BusCreator  Inputs=4
  Bus Selector : BusSelector  OutputSignals=controls_in.u_fuel,omega_engine_data_radS.omega_engine_data_radS,intake_man_out.p_in_man,exhaust_man_out.p_exh_man,intake_man_out.T_in_man,exhaust_man_out.T_exh_man
  Bus Selector1 : BusSelector  OutputSignals=controls_in.u_fuel,intake_man_out.F_in_man
  Bus Selector2 : BusSelector  OutputSignals=omega_engine_data_radS.omega_engine_data_radS,intake_man_out.T_in_man,controls_in.u_fuel,intake_man_out.F_in_man
  "Exhaust " : Subsystem
  Fcn : Fcn  Expr=(u(2)*u(3)+(1+14.6)*u(1))/(u(1)+u(3))
  Gain : Gain
  Mux : Mux  Inputs=3
  Saturation : Saturate  UpperLimit=1  LowerLimit=0
  Sum : Sum
  cylinder comp : Subsystem
  combustion_out : Outport
  W_cyl_sim : Outport  Port=2
  T_exhaust : Outport  Port=3
  W_engine_out : Outport  Port=4
  F_engine_out : Outport  Port=5
  sat_out-3 : Outport  Port=6
  wires:
  cylinder comp/1(W_cyl_sim) -> Gain/1  "W_cylinderr"
  "Exhaust "/1(T_exhaust) -> T_exhaust/1, Bus Creator/2  "T_exhaust"
  Bus Creator/1 -> combustion_out/1  "combustion_out"
  Omega_engine_radS/1 -> Bus Creator1/1
  intake_man_out/1 -> Bus Creator1/2
  exhaust_man_out/1 -> Bus Creator1/3
  controls_in/1 -> Bus Creator1/4
  Bus Creator1/1 -> Bus Selector/1, Bus Selector2/1, Bus Selector1/1
  Bus Selector/2 -> cylinder comp/1(omega_engine_radS)  "<omega_engine_data_radS>"
  Bus Selector/3 -> cylinder comp/2(p_intake_man)  "<p_in_man>"
  Bus Selector/4 -> cylinder comp/3(p_exhaust_man)  "<p_exh_man>"
  Bus Selector/5 -> cylinder comp/4(T_intake_man)  "<T_in_man>"
  Bus Selector/6 -> cylinder comp/5(T_exhaust_man)  "<T_exh_man>"
  Bus Selector2/1 -> "Exhaust "/1(omega_engine_radS)  "<omega_engine_data_radS>"
  Bus Selector2/3 -> "Exhaust "/4(u_fuel)  "<u_fuel>"
  Bus Selector2/4 -> "Exhaust "/5(F1_in_man)  "<F_in_man>"
  Bus Selector2/2 -> "Exhaust "/2(T_intake_man)  "<T_in_man>"
  Bus Selector/1 -> Sum/1  "<u_fuel>"
  Sum/1 -> W_engine_out/1, Bus Creator/4  "W_engine_out"
  Bus Selector1/1 -> Mux/1  "<u_fuel>"
  Bus Selector1/2 -> Mux/2  "<F_in_man>"
  Gain/1 -> "Exhaust "/3(W_cyl), Mux/3, Bus Creator/1, W_cyl_sim/1, Sum/2  "W_cylinder"
  Mux/1 -> Fcn/1
  Fcn/1 -> Saturation/1, sat_out-3/1  "F_engine_out1"
  Saturation/1 -> F_engine_out/1, Bus Creator/3  "F_engine_out"

== system KD_cl_harness_cl_ouports_added/Compressor ==
  ambient_in : Inport
  pre_throttle_out : Inport  Port=2
  Omega_turbo_radS : Inport  Port=3
  Bus Creator : BusCreator  Inputs=3
  Bus Creator1 : BusCreator  Inputs=3
  Bus Selector : BusSelector  OutputSignals=ambient_in.p_in_comp_data,pre_throttle_out.p_pre_throttle,ambient_in.T_in_comp_data,Omega_turbo_radS.Omega_turbo_radS
  Comp Map : Subsystem
  compressor_out : Outport
  W_comp_sim : Outport  Port=2
  T_out_comp_sim : Outport  Port=3
  Tq_comp_sim : Outport  Port=4
  wires:
  Comp Map/1(W_comp_sim) -> W_comp_sim/1, Bus Creator/1  "W_compressor"
  Comp Map/2(T_out_comp_sim) -> T_out_comp_sim/1, Bus Creator/2  "T_out_comp_sim"
  Bus Creator/1 -> compressor_out/1  "compressor_out"
  Comp Map/3(Tq_comp) -> Tq_comp_sim/1, Bus Creator/3  "Tq_comp_sim"
  ambient_in/1 -> Bus Creator1/1
  pre_throttle_out/1 -> Bus Creator1/2
  Omega_turbo_radS/1 -> Bus Creator1/3
  Bus Creator1/1 -> Bus Selector/1
  Bus Selector/1 -> Comp Map/1(p_in_comp)  "<p_in_comp_data>"
  Bus Selector/2 -> Comp Map/2(p_out_comp)  "<p_pre_throttle>"
  Bus Selector/3 -> Comp Map/3(T_in_comp_data)  "<T_in_comp_data>"
  Bus Selector/4 -> Comp Map/4(omega_turbo_data_radS)  "<Omega_turbo_radS>"

== system KD_cl_harness_cl_ouports_added/EGR Throttle ==
  controls_in : Inport
  Omega_engine_radS : Inport  Port=2
  intake_man_out : Inport  Port=3
  intercooler_out : Inport  Port=4
  p_preThrottle : Inport  Port=5
  Bus Creator : BusCreator  Inputs=1
  Bus Creator1 : BusCreator  Inputs=5
  Bus Selector : BusSelector  OutputSignals=controls_in.u_EGR_throttle,omega_engine_data_radS.omega_engine_data_radS,intake_man_out.p_in_man,intercooler_out.T_out_IC,pre_throttle_out.p_pre_throttle
  EGR Throttle : Subsystem
  egr_throttle_out : Outport
  W_EGR_Throttle : Outport  Port=2
  sat_out-6 : Outport  Port=3
  sat_out-37 : Outport  Port=4
  sat_out-38 : Outport  Port=5
  sat_out-39 : Outport  Port=6
  sat_out-40 : Outport  Port=7
  out-1 : Outport  Port=8
  out-3 : Outport  Port=9
  out-4 : Outport  Port=10
  wires:
  EGR Throttle/1(ThrottleFlow_kgpers) -> Bus Creator/1, W_EGR_Throttle/1  "W_EGR_Throttle"
  Bus Creator/1 -> egr_throttle_out/1  "egr_throttle_out"
  controls_in/1 -> Bus Creator1/1
  Omega_engine_radS/1 -> Bus Creator1/2
  intake_man_out/1 -> Bus Creator1/3
  intercooler_out/1 -> Bus Creator1/4
  Bus Creator1/1 -> Bus Selector/1
  Bus Selector/1 -> EGR Throttle/1(u_EGR_throttle)  "<u_EGR_throttle>"
  Bus Selector/2 -> EGR Throttle/2(omega_engine_radS)  "<omega_engine_data_radS>"
  Bus Selector/3 -> EGR Throttle/3(p_intake_man)  "<p_in_man>"
  Bus Selector/4 -> EGR Throttle/4(T_out_IC)  "<T_out_IC>"
  Bus Selector/5 -> EGR Throttle/5(p_preThrottle)  "<p_pre_throttle>"
  p_preThrottle/1 -> Bus Creator1/5
  EGR Throttle/2(sat_out-6) -> sat_out-6/1
  EGR Throttle/3(sat_out-37) -> sat_out-37/1
  EGR Throttle/4(sat_out-38) -> sat_out-38/1
  EGR Throttle/5(sat_out-39) -> sat_out-39/1
  EGR Throttle/6(sat_out-40) -> sat_out-40/1
  EGR Throttle/7(out-1) -> out-1/1
  EGR Throttle/8(out-3) -> out-3/1
  EGR Throttle/9(out-4) -> out-4/1

== system KD_cl_harness_cl_ouports_added/EGR Valve ==
  controls_in : Inport
  omega_engine_data_radS : Inport  Port=2
  intake_man_out : Inport  Port=3
  exhaust_man_out : Inport  Port=4
  egr_cooler_out : Inport  Port=5
  Bus Creator : BusCreator  Inputs=1
  Bus Creator1 : BusCreator  Inputs=5
  Bus Selector : BusSelector  OutputSignals=controls_in.u_EGR_valve,omega_engine_data_radS.omega_engine_data_radS,intake_man_out.p_in_man,egr_cooler_out.T_out_EGR_cooler,exhaust_man_out.p_exh_man
  SVR EGR : Subsystem
  egr_valve_out : Outport
  W_EGR_out : Outport  Port=2
  sat_out-41 : Outport  Port=3
  sat_out-42 : Outport  Port=4
  sat_out-43 : Outport  Port=5
  sat_out-44 : Outport  Port=6
  out-2 : Outport  Port=7
  out-5 : Outport  Port=8
  out-6 : Outport  Port=9
  wires:
  SVR EGR/1(EGR_kgpers) -> Bus Creator/1, W_EGR_out/1  "W_EGR_valve"
  Bus Creator/1 -> egr_valve_out/1  "egr_valve_out"
  controls_in/1 -> Bus Creator1/1
  omega_engine_data_radS/1 -> Bus Creator1/2
  intake_man_out/1 -> Bus Creator1/3
  exhaust_man_out/1 -> Bus Creator1/4
  Bus Creator1/1 -> Bus Selector/1
  Bus Selector/1 -> SVR EGR/1(u_EGR_valve)  "<u_EGR_valve>"
  Bus Selector/2 -> SVR EGR/2(omega_engine_data_radS)  "<omega_engine_data_radS>"
  Bus Selector/3 -> SVR EGR/3(p_intake_man_data)  "<p_in_man>"
  Bus Selector/4 -> SVR EGR/4(T_out_egr_cooler)  "<T_out_EGR_cooler>"
  Bus Selector/5 -> SVR EGR/5(p_exhaust_man_data)  "<p_exh_man>"
  egr_cooler_out/1 -> Bus Creator1/5
  SVR EGR/2(sat_out-41) -> sat_out-41/1
  SVR EGR/3(sat_out-42) -> sat_out-42/1
  SVR EGR/4(sat_out-43) -> sat_out-43/1
  SVR EGR/5(sat_out-44) -> sat_out-44/1
  SVR EGR/6(out-2) -> out-2/1
  SVR EGR/7(out-5) -> out-5/1
  SVR EGR/8(out-6) -> out-6/1

== system KD_cl_harness_cl_ouports_added/EGR cooler ==
  note: Estimation of T_in_egr cooler is to be done
      | as T_exh_man and T_in_egr_cooler are
      | significantly different
  T_exh_man : Inport
  ambient_in : Inport  Port=2
  egr_valve_out : Inport  Port=3
  controls_in : Inport  Port=4
  Omega_engine_radS : Inport  Port=5
  Bus Creator : BusCreator  Inputs=2
  Bus Creator1 : BusCreator  Inputs=5
  Bus Selector : BusSelector  OutputSignals=exhaust_man_out.T_exh_man,ambient_in.T_coolant,egr_valve_out.W_EGR_valve,controls_in.u_EGR_cooler_bypass,omega_engine_data_radS.omega_engine_data_radS,ambient_in.T_ambient
  EGR Cooler : Subsystem
  egr_cooler_out : Outport
  T_out_EGR_cooler : Outport  Port=2
  wires:
  EGR Cooler/1(T_out_EGR_cooler_sim) -> Bus Creator/1, T_out_EGR_cooler/1  "T_out_EGR_cooler"
  Bus Creator/1 -> egr_cooler_out/1  "egr_cooler_out"
  Bus Creator1/1 -> Bus Selector/1
  Bus Selector/1 -> EGR Cooler/1(T_exh_man)  "<T_exh_man>"
  Bus Selector/2 -> EGR Cooler/2(T_coolant)  "<T_coolant>"
  Bus Selector/3 -> EGR Cooler/3(W_egr_valve)  "<W_EGR_valve>"
  Bus Selector/4 -> EGR Cooler/4(u_EGR_cooler_bypass)  "<u_EGR_cooler_bypass>"
  Bus Selector/5 -> EGR Cooler/5(omega_engine_data_radS)  "<omega_engine_data_radS>"
  EGR Cooler/2(W_egr_cooler) -> Bus Creator/2  "W_egr_cooler"
  Bus Selector/6 -> EGR Cooler/6(T_ambient)  "<T_ambient>"
  T_exh_man/1 -> Bus Creator1/1
  ambient_in/1 -> Bus Creator1/2
  egr_valve_out/1 -> Bus Creator1/3
  controls_in/1 -> Bus Creator1/4
  Omega_engine_radS/1 -> Bus Creator1/5

== system KD_cl_harness_cl_ouports_added/Exhaust Manifold ==
  egr_valve_out : Inport
  controls_in : Inport  Port=2
  turbine_out : Inport  Port=3
  combustion_out : Inport  Port=4
  intake_man_out : Inport  Port=5
  ambient_in : Inport  Port=6
  Bus Creator : BusCreator  Inputs=3
  Bus Creator1 : BusCreator  Inputs=6
  Bus Selector : BusSelector  OutputSignals=egr_valve_out.W_EGR_valve,combustion_out.W_cylinder,controls_in.u_fuel,turbine_out.W_turbine,combustion_out.F_engine_out,combustion_out.T_exhaust,intake_man_out.T_in_man,ambient_in.T_ambient
  Exhaust Manifold : Subsystem
  exhaust_man_out : Outport
  p_exh_man_sim : Outport  Port=2
  T_exh_man_sim : Outport  Port=3
  F_exh_man_sim : Outport  Port=4
  wires:
  Exhaust Manifold/1(p_exh_man_sim) -> p_exh_man_sim/1, Bus Creator/1  "p_exh_man"
  Exhaust Manifold/2(T_exh_man_sim) -> T_exh_man_sim/1, Bus Creator/2  "T_exh_man"
  Exhaust Manifold/3(F_exh_man_sim) -> F_exh_man_sim/1, Bus Creator/3  "F_exh_man"
  Bus Creator/1 -> exhaust_man_out/1  "exhaust_man_out"
  Bus Creator1/1 -> Bus Selector/1
  Bus Selector/3 -> Exhaust Manifold/3(u_fuel)  "<u_fuel>"
  Bus Selector/4 -> Exhaust Manifold/4(W_turbine)  "<W_turbine>"
  Bus Selector/5 -> Exhaust Manifold/5(F_engine_out)  "<F_engine_out>"
  Bus Selector/6 -> Exhaust Manifold/6(exhaust_temp)  "<T_exhaust>"
  egr_valve_out/1 -> Bus Creator1/1
  controls_in/1 -> Bus Creator1/2
  turbine_out/1 -> Bus Creator1/3
  combustion_out/1 -> Bus Creator1/4
  Bus Selector/1 -> Exhaust Manifold/1(W_egr_valve)  "<W_EGR_valve>"
  Bus Selector/2 -> Exhaust Manifold/2(W_cylinder)  "<W_cylinder>"
  intake_man_out/1 -> Bus Creator1/5
  Bus Selector/7 -> Exhaust Manifold/7(T_intake_man)  "<T_in_man>"
  ambient_in/1 -> Bus Creator1/6
  Bus Selector/8 -> Exhaust Manifold/8(T_ambient)  "<T_ambient>"

== system KD_cl_harness_cl_ouports_added/Intake Manifold ==
  throttle_out : Inport
  egr_cooler_out : Inport  Port=2
  exhaust_man_out : Inport  Port=3
  intecooler_out : Inport  Port=4
  combustion_out : Inport  Port=5
  Bus Creator : BusCreator  Inputs=3
  Bus Creator1 : BusCreator  Inputs=5
  Bus Selector : BusSelector  OutputSignals=egr_throttle_out.W_EGR_Throttle,egr_cooler_out.W_egr_cooler,combustion_out.W_cylinder,exhaust_man_out.F_exh_man,egr_cooler_out.T_out_EGR_cooler,intercooler_out.T_out_IC
  Intake_manifold : Subsystem
  intake_man_out : Outport
  p_in_man_sim : Outport  Port=2
  T_in_man_sim : Outport  Port=3
  F_in_man_sim : Outport  Port=4
  wires:
  Intake_manifold/1(p_in_man_sim) -> p_in_man_sim/1, Bus Creator/1  "p_in_man"
  Intake_manifold/2(T_in_man_sim) -> T_in_man_sim/1, Bus Creator/2  "T_in_man"
  Intake_manifold/3(F_in_man_sim) -> F_in_man_sim/1, Bus Creator/3  "F_in_man"
  Bus Creator/1 -> intake_man_out/1  "intake_man_out"
  throttle_out/1 -> Bus Creator1/1
  egr_cooler_out/1 -> Bus Creator1/2
  exhaust_man_out/1 -> Bus Creator1/3
  Bus Creator1/1 -> Bus Selector/1
  Bus Selector/1 -> Intake_manifold/1(W_throttle)  "<W_EGR_Throttle>"
  Bus Selector/2 -> Intake_manifold/2(W_egr_valve)  "<W_egr_cooler>"
  Bus Selector/4 -> Intake_manifold/4(F2_exhaust_sim)  "<F_exh_man>"
  Bus Selector/5 -> Intake_manifold/5(T_out_egr_cooler)  "<T_out_EGR_cooler>"
  intecooler_out/1 -> Bus Creator1/4
  Bus Selector/6 -> Intake_manifold/6(T_out_IC)  "<T_out_IC>"
  combustion_out/1 -> Bus Creator1/5
  Bus Selector/3 -> Intake_manifold/3(W_cyl_in)  "<W_cylinder>"

== system KD_cl_harness_cl_ouports_added/Intercooler ==
  compressor_out : Inport
  pre_throttle_out : Inport  Port=2
  T_ambient : Inport  Port=3
  Bus Creator : BusCreator  Inputs=3
  Bus Creator1 : BusCreator  Inputs=2
  Bus Selector : BusSelector  OutputSignals=compressor_out.T_out_comp_sim,pre_throttle_out.p_pre_throttle,ambient_in.T_ambient
  Intercooler : Subsystem
  intercooler_out : Outport
  T_out_IC : Outport  Port=2
  wires:
  compressor_out/1 -> Bus Creator/1
  pre_throttle_out/1 -> Bus Creator/2
  Bus Creator/1 -> Bus Selector/1
  Bus Selector/1 -> Intercooler/1(T_out_comp)  "<T_out_comp_sim>"
  Bus Selector/2 -> Intercooler/2(p_out_comp)  "<p_pre_throttle>"
  Intercooler/1(T_out_IC) -> Bus Creator1/1, T_out_IC/1  "T_out_IC"
  Intercooler/2(p_out_IC) -> Bus Creator1/2  "p_out_IC"
  Bus Creator1/1 -> intercooler_out/1  "intercooler_out"
  T_ambient/1 -> Bus Creator/3
  Bus Selector/3 -> Intercooler/3(T_ambient)  "<T_ambient>"

== system KD_cl_harness_cl_ouports_added/NEDC_cycle ==
  From Workspace1 : FromWorkspace  VariableName=[ECUTIME s2g_eqfine_eqfine]  SampleTime=sample_time  Interpolate=off  OutputAfterFinalValue=Holding final value
  From Workspace3 : FromWorkspace  VariableName=[ECUTIME s2g_ene_ene]  SampleTime=sample_time  Interpolate=off  OutputAfterFinalValue=Holding final value
  Mux3 : Mux  Inputs=2
  Saturation : Saturate  UpperLimit=inf  LowerLimit=750
      settings: AttributesFormatString=%<LowerLimit>\n%<UpperLimit>
  Saturation1 : Saturate  UpperLimit=inf  LowerLimit=0
      settings: AttributesFormatString=%<LowerLimit>\n%<UpperLimit>
  Subsystem1 : Subsystem  TreatAsAtomicUnit=on  SystemSampleTime=.032
  Out1 : Outport
  sat_out-4 : Outport  Port=2
  sat_out-5 : Outport  Port=3
  wires:
  From Workspace3/1 -> Saturation/1, sat_out-4/1
  From Workspace1/1 -> Saturation1/1, sat_out-5/1
  Saturation1/1 -> Mux3/1
  Saturation/1 -> Subsystem1/1(In1)
  Mux3/1 -> Out1/1
  Subsystem1/1(Out1) -> Mux3/2

== system KD_cl_harness_cl_ouports_added/Turbine ==
  omega_turbo_radS : Inport
  exhaust_man_out : Inport  Port=2
  ambient_In : Inport  Port=3
  controls_In : Inport  Port=4
  Bus Creator : BusCreator  Inputs=3
  Bus Creator1 : BusCreator  Inputs=4
  Bus Selector : BusSelector  OutputSignals=Omega_turbo_radS.Omega_turbo_radS,exhaust_man_out.p_exh_man,ambient_in.T_ambient,exhaust_man_out.T_exh_man,controls_in.u_VGT
  TurbineMap : Subsystem
  turbine_out : Outport
  W_out_turb_sim : Outport  Port=2
  T_out_turb_sim : Outport  Port=3
  Tq_turbine : Outport  Port=4
  wires:
  TurbineMap/1(W_out_turb_sim) -> W_out_turb_sim/1, Bus Creator/1  "W_turbine"
  TurbineMap/2(T_out_turb_sim) -> T_out_turb_sim/1, Bus Creator/2  "T_out_turbine"
  Bus Creator/1 -> turbine_out/1  "turbine_out"
  TurbineMap/3(Tq_turbine) -> Tq_turbine/1, Bus Creator/3  "Tq_turbine"
  omega_turbo_radS/1 -> Bus Creator1/1
  exhaust_man_out/1 -> Bus Creator1/2
  ambient_In/1 -> Bus Creator1/3
  controls_In/1 -> Bus Creator1/4
  Bus Creator1/1 -> Bus Selector/1
  Bus Selector/3 -> TurbineMap/3(T_ambient)  "<T_ambient>"
  Bus Selector/4 -> TurbineMap/4(T_exhaust_man)  "<T_exh_man>"
  Bus Selector/5 -> TurbineMap/5(u_VGT)  "<u_VGT>"
  Bus Selector/1 -> TurbineMap/1(omega_turbo_radS)  "<Omega_turbo_radS>"
  Bus Selector/2 -> TurbineMap/2(p_exhaust_man)  "<p_exh_man>"

== system KD_cl_harness_cl_ouports_added/Turbo Rotational Dynamics ==
  compressor_out : Inport
  turbine_out : Inport  Port=2
  Bus Creator : BusCreator  Inputs=1
  Bus Creator1 : BusCreator  Inputs=2
  Bus Selector : BusSelector  OutputSignals=compressor_out.Tq_comp_sim,turbine_out.Tq_turbine
  Turbo rot : Subsystem
  Omega_turbo_radS : Outport
  Omega_turbo_out_radS : Outport  Port=2
  wires:
  Turbo rot/1(Omega_turbo_radS) -> Omega_turbo_out_radS/1, Bus Creator/1  "Omega_turbo_radS"
  Bus Creator/1 -> Omega_turbo_radS/1  "Omega_turbo_radS"
  compressor_out/1 -> Bus Creator1/1
  turbine_out/1 -> Bus Creator1/2
  Bus Creator1/1 -> Bus Selector/1
  Bus Selector/1 -> Turbo rot/1(Tq_compressor)  "<Tq_comp_sim>"
  Bus Selector/2 -> Turbo rot/2(Tq_turbine)  "<Tq_turbine>"
